simulink model "test_continuous_ss_lpv_model"  (R2020a)
settings: Solver=FixedStepAuto  StartTime=0.0  StopTime=t(end)  FixedStep=Ts  RelTol=1e-3
values from neighbouring files (symbols this model uses):
  A0 = T*A0*inv(T)    [test_continuous_ss_lpv.m]    (also in test_continuous_ss_tv.m; test_discrete_ss_lpv.m; test_discrete_ss_tv.m)
  A1 = 1e-10*round(2*(rand(n,n)-0.5))    [test_continuous_ss_lpv.m]    (also in test_continuous_ss_tv.m; test_discrete_ss_lpv.m; test_discrete_ss_tv.m)
  B0 = rand(n,m)    [test_continuous_ss_lpv.m]    (also in test_continuous_ss_tv.m; test_discrete_ss_lpv.m; test_discrete_ss_tv.m)
  B1 = 1e-3*round(2*(rand(n,m)-0.5))    [test_continuous_ss_lpv.m]    (also in test_continuous_ss_tv.m = round(2*(rand(n,m)-0.5)); test_discrete_ss_lpv.m; test_discrete_ss_tv.m = round(2*(rand(n,m)-0.5)))
  C0 = rand(p,n)    [test_continuous_ss_lpv.m]    (also in test_continuous_ss_tv.m; test_discrete_ss_lpv.m; test_discrete_ss_tv.m)
  C1 = 1e-3*round(2*(rand(p,n)-0.5))    [test_continuous_ss_lpv.m]    (also in test_continuous_ss_tv.m = round(2*(rand(p,n)-0.5)); test_discrete_ss_lpv.m; test_discrete_ss_tv.m = round(2*(rand(p,n)-0.5)))
  D0 = rand(p,m)    [test_continuous_ss_lpv.m]    (also in test_continuous_ss_tv.m; test_discrete_ss_lpv.m; test_discrete_ss_tv.m)
  D1 = 1e-3*round(2*(rand(p,m)-0.5))    [test_continuous_ss_lpv.m]    (also in test_continuous_ss_tv.m = round(2*(rand(p,m)-0.5)); test_discrete_ss_lpv.m; test_discrete_ss_tv.m = round(2*(rand(p,m)-0.5)))
  initial_state = rand(n,1)    [test_continuous_ss_lpv.m]    (also in test_continuous_ss_ti.m; test_continuous_ss_tv.m; test_discrete_ss_lpv.m; test_discrete_ss_ti.m)
  Ts = 0.001    [test_PIDISA_controller.m]    (also in test_PID_controller.m; test_continuous_ss_lpv.m = 0.0001; test_continuous_ss_ti.m = 0.0001; test_continuous_ss_tv.m = 0.0001)
undefined symbols (not defined in the file or in its folder): Ap, Bp, Cp, Dp
settings Model: Creator=bascetta  LastModifiedBy=bascetta
settings DataIOCC: SaveOutput=off  SignalLogging=off  DSMLogging=off  SaveTime=off

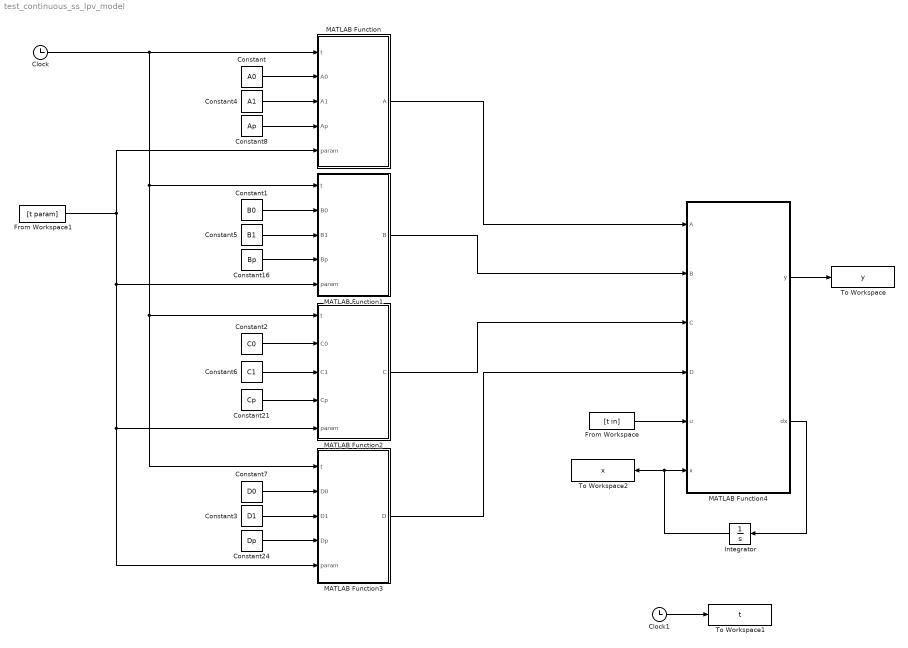
== system test_continuous_ss_lpv_model ==
  Clock : Clock
  Clock1 : Clock
  Constant : Constant  Value=A0  VectorParams1D=off
  Constant1 : Constant  Value=B0  VectorParams1D=off
  Constant16 : Constant  Value=Bp  VectorParams1D=off
  Constant2 : Constant  Value=C0  VectorParams1D=off
  Constant21 : Constant  Value=Cp  VectorParams1D=off
  Constant24 : Constant  Value=Dp  VectorParams1D=off
  Constant3 : Constant  Value=D1  VectorParams1D=off
  Constant4 : Constant  Value=A1  VectorParams1D=off
  Constant5 : Constant  Value=B1  VectorParams1D=off
  Constant6 : Constant  Value=C1  VectorParams1D=off
  Constant7 : Constant  Value=D0  VectorParams1D=off
  Constant8 : Constant  Value=Ap  VectorParams1D=off
  From Workspace : FromWorkspace  VariableName=[t in]  SampleTime=Ts
  From Workspace1 : FromWorkspace  VariableName=[t param]  SampleTime=Ts
  Integrator : Integrator  InitialCondition=initial_state
  MATLAB Function : MATLAB Function  TreatAsAtomicUnit=on
  MATLAB Function1 : MATLAB Function  TreatAsAtomicUnit=on
  MATLAB Function2 : MATLAB Function  TreatAsAtomicUnit=on
  MATLAB Function3 : MATLAB Function  TreatAsAtomicUnit=on
  MATLAB Function4 : MATLAB Function  TreatAsAtomicUnit=on
  To Workspace : ToWorkspace  VariableName=y  SampleTime=Ts
      settings: Save2DSignal=2-D array (concatenate along first dimension)
  To Workspace1 : ToWorkspace  VariableName=t  SampleTime=Ts
      settings: Save2DSignal=2-D array (concatenate along first dimension)
  To Workspace2 : ToWorkspace  VariableName=x  SampleTime=Ts
      settings: Save2DSignal=2-D array (concatenate along first dimension)
  wires:
  From Workspace/1 -> MATLAB Function4/5(u)
  MATLAB Function4/1(y) -> To Workspace/1
  MATLAB Function4/2(dx) -> Integrator/1
  Integrator/1 -> To Workspace2/1, MATLAB Function4/6(x)
  Clock1/1 -> To Workspace1/1
  Constant/1 -> MATLAB Function/2(A0)
  Constant4/1 -> MATLAB Function/3(A1)
  Constant1/1 -> MATLAB Function1/2(B0)
  Constant5/1 -> MATLAB Function1/3(B1)
  Constant2/1 -> MATLAB Function2/2(C0)
  Constant6/1 -> MATLAB Function2/3(C1)
  Constant7/1 -> MATLAB Function3/2(D0)
  Constant3/1 -> MATLAB Function3/3(D1)
  Constant8/1 -> MATLAB Function/4(Ap)
  Constant16/1 -> MATLAB Function1/4(Bp)
  Constant21/1 -> MATLAB Function2/4(Cp)
  Constant24/1 -> MATLAB Function3/4(Dp)
  Clock/1 -> MATLAB Function2/1(t), MATLAB Function3/1(t), MATLAB Function1/1(t), MATLAB Function/1(t)
  From Workspace1/1 -> MATLAB Function2/5(param), MATLAB Function3/5(param), MATLAB Function1/5(param), MATLAB Function/5(param)
  MATLAB Function/1(A) -> MATLAB Function4/1(A)
  MATLAB Function1/1(B) -> MATLAB Function4/2(B)
  MATLAB Function2/1(C) -> MATLAB Function4/3(C)
  MATLAB Function3/1(D) -> MATLAB Function4/4(D)

== matlab function test_continuous_ss_lpv_model/MATLAB Function1 ==
  data: t input; B output; B0 input; B1 input; Bp input; param input
function B = B_matrix(t,B0,B1,Bp,param)

B = B0+B1*(t^0.5);

for i=1:length(param)
    B = B+Bp(:,:,i)*param(i);
end

== matlab function test_continuous_ss_lpv_model/MATLAB Function ==
  data: t input; A output; A0 input; A1 input; Ap input; param input
function A = A_matrix(t,A0,A1,Ap,param)

A = A0+A1*(t^0.5);

for i=1:length(param)
    A = A+Ap(:,:,i)*param(i);
end

== matlab function test_continuous_ss_lpv_model/MATLAB Function2 ==
  data: t input; C output; C0 input; C1 input; Cp input; param input
function C = C_matrix(t,C0,C1,Cp,param)

C = C0+C1*(t^0.5);

for i=1:length(param)
    C = C+Cp(:,:,i)*param(i);
end

== matlab function test_continuous_ss_lpv_model/MATLAB Function3 ==
  data: t input; D output; D0 input; D1 input; Dp input; param input
function D = D_matrix(t,D0,D1,Dp,param)

D = D0+D1*(t^0.5);

for i=1:length(param)
    D = D+Dp(:,:,i)*param(i);
end

== matlab function test_continuous_ss_lpv_model/MATLAB Function4 ==
  data: A input; B input; C input; D input; u input; x input; y output; dx output
function [y,dx] = statespace_model(A,B,C,D,u,x)

dx = zeros(size(A,1),1);
y  = zeros(size(C,1),1);

dx = A*x+B*u;
y  = C*x+D*u;
